simulink model "fuzblkrule"  (Simulink 2.20)
settings: Solver=ode45  StartTime=0.0  StopTime=10.0  RelTol=1e-3  AbsTol=1e-6
settings Model: ConsistencyChecking=off  RTWPlaceOutputsASAP=off  RTWTemplateMakefile=grt_unix.tmf

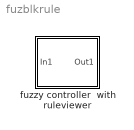
== system fuzblkrule ==
  fuzzy controller  with ruleviewer : Subsystem
      mask Type: FIS
      mask Display: plot(0, -0.3, 6, -0.3, 0, 1.2, 6, 1.2, [0 6], [0 0], [1 2 3],[0 1 0],[2 3 4],[0 1 0],[3 4 5],[0 1 0])

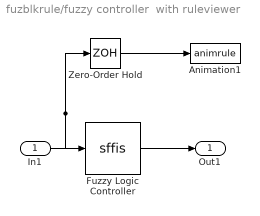
== system fuzblkrule/fuzzy controller  with ruleviewer ==
  In1 : Inport  Port=1  PortWidth=-1  SampleTime=-1
  Animation1 : S-Function  FunctionName=animrule  Parameters=fismatrix  PortCounts=[]  SFunctionModules=''
  Fuzzy Logic Controller : S-Function  FunctionName=sffis  Parameters=fismatrix  PortCounts=[]  SFunctionModules=sfsup  mask(FIS){@1=fismat}
      mask prompts: @1 "FIS Matrix:"
      mask help: FIS
      mask init:
      | fismatrix = @1;
      mask Help: Fuzzy Inference System
      mask Display: plot(0, -0.3, 6, -0.3, 0, 1.2, 6, 1.2, [0 6], [0 0], [1 2 3],[0 1 0],[2 3 4],[0 1 0],[3 4 5],[0 1 0])
  Zero-Order Hold : ZeroOrderHold  SampleTime=2
  Out1 : Outport  Port=1  InitialOutput=0
  wires:
  In1/1 -> Fuzzy Logic Controller/1, Zero-Order Hold/1
  Fuzzy Logic Controller/1 -> Out1/1
  Zero-Order Hold/1 -> Animation1/1
